simulink model "trim_cessna_t37"  (Simulink 9.0)
settings: Solver=ode45  StartTime=0.0  StopTime=10.0  RelTol=1e-3  EnableMultiTasking=on
values from neighbouring files (symbols this model uses):
  Aero_RP = Aero_RP*[-1 0 0;0 1 0;0 0 -1]    [t37_data.m]
  aileron_limits = [-0.35 0.35]*pi/180    [t37_data.m]
  CD_alpha = 0.3840    (= 0.384)    [t37_data.m]
  CD_beta = [-1.5700	1.2300 ... (first row only)    [t37_data.m]
  CD_de = 0.0750    (= 0.075)    [t37_data.m]
  CD_flap = 0.0750    (= 0.075)    [t37_data.m]
  CD_ground_effect = [0.0000	0.8100 ... (first row only)    [t37_data.m]
  CD_zero = [  -1.5700	1.5000 ... (first row only)    [t37_data.m]
  Cl_ail = [0.0000	0.1810 ... (first row only)    [t37_data.m]
  CL_alpha = [-0.2000	-0.6400 ... (first row only)    [t37_data.m]
  CL_alpha_dot = 2.0    (= 2)    [t37_data.m]
  Cl_beta = -0.0944    [t37_data.m]
  CL_elev = 0.5    [t37_data.m]
  CL_flap = 0.3500    (= 0.35)    [t37_data.m]
  CL_ground_effect = [0.0000	1.0610 ... (first row only)    [t37_data.m]
  Cl_p = -0.4420    (= -0.442)    [t37_data.m]
  CL_q = 4.1    [t37_data.m]
  Cl_r = 0.0926    [t37_data.m]
  Cl_rudder = 0.0150    (= 0.015)    [t37_data.m]
  Cm_alpha = -0.7000    (= -0.7)    [t37_data.m]
  Cm_alpha_dot = -6.9500    (= -6.95)    [t37_data.m]
  Cm_elev = [0.0000	-1.1200 ... (first row only)    [t37_data.m]
  Cm_q = -50.0000    (= -50)    [t37_data.m]
  Cm_zero = 0.0250    (= 0.025)    [t37_data.m]
  Cn_beta = 0.1106    [t37_data.m]
  Cn_p = -0.0243    [t37_data.m]
  Cn_r = -0.1390    (= -0.139)    [t37_data.m]
  Cn_rudder = -0.0365    [t37_data.m]
  Cnda = -0.0254    [t37_data.m]
  CY_beta = -0.3460    (= -0.346)    [t37_data.m]
  CY_p = -0.0827    [t37_data.m]
  CY_r = 0.3000    (= 0.3)    [t37_data.m]
  CY_rudder = 0.200    (= 0.2)    [t37_data.m]
  elevator_limits = [-0.35 0.3]*pi/180    [t37_data.m]
  isTrimming = 0    [mytrim.m]    (also in t37_data.m)
  Jxx = 7985*1.3558179    (= 10826.2059315)    [t37_data.m]
  Jxz = 0    [t37_data.m]
  Jyy = 6000*1.3558179    (= 8134.9074)    [t37_data.m]
  Jzz = 11183*1.3558179    (= 15162.1115757)    [t37_data.m]
  M = 4056*0.45359237    (= 1839.77065272)    [t37_data.m]
  Rcg = Rcg*[-1 0 0;0 1 0;0 0 -1]    [t37_data.m]
  Rengine1 = Rengine1*[-1 0 0;0 1 0;0 0 -1]    [t37_data.m]
  Rengine2 = Rengine2*[-1 0 0;0 1 0;0 0 -1]    [t37_data.m]
  rudder_limits = [-0.35 0.35]*pi/180    [t37_data.m]
  Sw = 182*0.09290304    (= 16.90835328)    [t37_data.m]
  thrust_limits = [0 1]    [t37_data.m]
  Tmax = M*10    (= 18397.7065272)    [t37_data.m]
undefined symbols (not defined in the file or in its folder): CD_mach, DCnpDf
undefined symbols (not defined in the file): Bw, Cw
libraries: sharedutil x1
(part 1 of 2)
settings Model: Creator=torres  LastModifiedBy=Pc melhor q do euler  ExtModeAutoUpdateStatusClock=off
settings DataIOCC: LimitDataPoints=on  SignalLoggingSaveFormat=ModelDataLogs  SignalLoggingName=sigsOut
settings DebuggingCC: SaveWithParameterizedLinksMsg=none  SignalResolutionControl=TryResolveAllWithWarning  MultiTaskDSMMsg=warning  MultiTaskCondExecSysMsg=none  FcnCallInpInsideContextMsg=warning  StrictBusMsg=None
settings HardwareCC: TargetHWDeviceType=32-bit Generic  TargetUnknown=on  ProdEqTarget=off
settings GRTTargetCC: TargetFcnLib=ansi_tfl_tmw.mat  CombineOutputUpdateFcns=off  GRTInterface=on

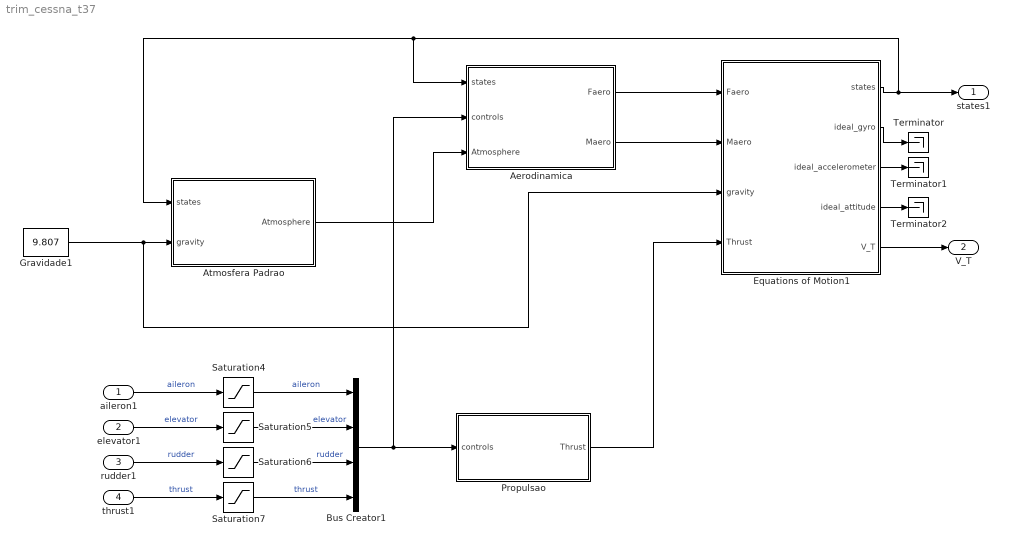
== system trim_cessna_t37 ==
  aileron1 : Inport
  elevator1 : Inport  Port=2
  rudder1 : Inport  Port=3
  thrust1 : Inport  Port=4
  Aerodinamica : Subsystem  mask{flap=0, bw=Bw, cw=Cw, Sw=Sw}
      mask prompts: flap "Comando Flap (0, 1, 2 ou 3)"; bw "Comprimento da asa  - wingspan (m)"; cw "Corda media da asa (m)"; Sw "Area da asa (m2)"
  Atmosfera Padrao : Subsystem
  Bus Creator1 : BusCreator  Inputs=4
  Equations of Motion1 : Subsystem  mask{R_engine=Rengine1, Rcg=Rcg, Aero_RP=Aero_RP, m=M, Jxz=Jxz, Jxx=Jxx, Jyy=Jyy, Jzz=Jzz, d=[0; 0; 0]}
      mask prompts: R_engine "Engine position (row vector in meters)"; Rcg "C.G. position (m)"; Aero_RP "Nominal C.G. (m) = Aerodynamic Reference Point"; m "Aircraft mass (Kg)"; Jxz "Inertia product (Jxz)"; Jxx "Inertia (Jxx)"; Jyy "Inertia (Jyy)"; Jzz "Inertia (Jzz)"; d "Accelerometers displacement from CG (vector in the ABC frame, in (m))"
  Gravidade1 : Constant  Value=9.807
  Propulsao : Subsystem  mask{Tmax=Tmax}
      mask prompts: Tmax "Tracao Maxima (N)"
  Saturation4 : Saturate  UpperLimit=aileron_limits(2)  LowerLimit=aileron_limits(1)
  Saturation5 : Saturate  UpperLimit=elevator_limits(2)  LowerLimit=elevator_limits(1)
  Saturation6 : Saturate  UpperLimit=rudder_limits(2)  LowerLimit=rudder_limits(1)
  Saturation7 : Saturate  UpperLimit=thrust_limits(2)  LowerLimit=thrust_limits(1)
  Terminator : Terminator
  Terminator1 : Terminator
  Terminator2 : Terminator
  states1 : Outport
  V_T : Outport  Port=2
  wires:
  Atmosfera Padrao/1(Atmosphere) -> Aerodinamica/3(Atmosphere)
  Equations of Motion1/1(states) -> Atmosfera Padrao/1(states), Aerodinamica/1(states), states1/1
  aileron1/1 -> Saturation4/1  "aileron"
  elevator1/1 -> Saturation5/1  "elevator"
  rudder1/1 -> Saturation6/1  "rudder"
  Gravidade1/1 -> Atmosfera Padrao/2(gravity), Equations of Motion1/3(gravity)
  thrust1/1 -> Saturation7/1  "thrust"
  Bus Creator1/1 -> Propulsao/1(controls), Aerodinamica/2(controls)
  Aerodinamica/1(Faero) -> Equations of Motion1/1(Faero)
  Aerodinamica/2(Maero) -> Equations of Motion1/2(Maero)
  Propulsao/1(Thrust) -> Equations of Motion1/4(Thrust)
  Saturation4/1 -> Bus Creator1/1  "aileron"
  Saturation5/1 -> Bus Creator1/2  "elevator"
  Saturation6/1 -> Bus Creator1/3  "rudder"
  Saturation7/1 -> Bus Creator1/4  "thrust"
  Equations of Motion1/2(ideal_gyro) -> Terminator/1
  Equations of Motion1/3(ideal_accelerometer) -> Terminator1/1
  Equations of Motion1/4(ideal_attitude) -> Terminator2/1
  Equations of Motion1/5(V_T) -> V_T/1

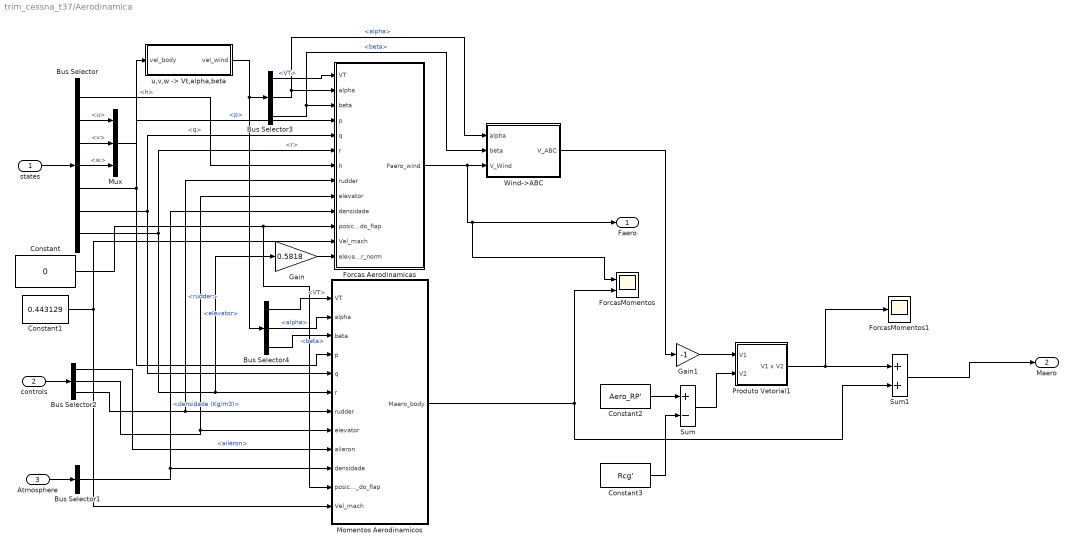
== system trim_cessna_t37/Aerodinamica ==
  states : Inport
  controls : Inport  Port=2
  Atmosphere : Inport  Port=3
  Bus Selector : BusSelector  OutputSignals=h,u,v,w,p,q,r
  Bus Selector1 : BusSelector  OutputSignals=densidade (Kg/m3)
  Bus Selector2 : BusSelector  OutputSignals=aileron,elevator,rudder
  Bus Selector3 : BusSelector  OutputSignals=VT,alpha,beta
  Bus Selector4 : BusSelector  OutputSignals=VT,alpha,beta
  Constant : Constant  Value=0
  Constant1 : Constant  Value=0.443129
  Constant2 : Constant  Value=Aero_RP'
  Constant3 : Constant  Value=Rcg'
  Forcas Aerodinamicas : Subsystem
  ForcasMomentos : Scope  NumInputPorts=2
  ForcasMomentos1 : Scope
  Gain : Gain  Gain=0.5818
  Gain1 : Gain  Gain=-1
  Momentos Aerodinamicos : Subsystem
  Mux : Mux  Inputs=3
  Produto Vetorial1 : Subsystem
  Sum : Sum  Inputs=+-  SaturateOnIntegerOverflow=on
  Sum1 : Sum  SaturateOnIntegerOverflow=on
  Wind->ABC : Subsystem
  "u,v,w -> Vt,alpha,beta" : Subsystem
  Faero : Outport
  Maero : Outport  Port=2
  wires:
  states/1 -> Bus Selector/1
  Atmosphere/1 -> Bus Selector1/1
  Bus Selector1/1 -> Momentos Aerodinamicos/10(densidade), Forcas Aerodinamicas/10(densidade)  "<densidade (Kg/m3)>"
  Bus Selector/1 -> Forcas Aerodinamicas/7(h)  "<h>"
  Bus Selector/5 -> Momentos Aerodinamicos/4(p), Forcas Aerodinamicas/4(p)  "<p>"
  Bus Selector/6 -> Momentos Aerodinamicos/5(q), Forcas Aerodinamicas/5(q)  "<q>"
  Bus Selector/7 -> Gain/1, Momentos Aerodinamicos/6(r), Forcas Aerodinamicas/6(r)  "<r>"
  controls/1 -> Bus Selector2/1
  Bus Selector2/1 -> Momentos Aerodinamicos/9(aileron)  "<aileron>"
  Bus Selector2/2 -> Momentos Aerodinamicos/8(elevator), Forcas Aerodinamicas/9(elevator)  "<elevator>"
  Bus Selector2/3 -> Momentos Aerodinamicos/7(rudder), Forcas Aerodinamicas/8(rudder)  "<rudder>"
  Bus Selector3/1 -> Forcas Aerodinamicas/1(VT)  "<VT>"
  Bus Selector3/2 -> Forcas Aerodinamicas/2(alpha), Wind->ABC/1(alpha)  "<alpha>"
  Bus Selector3/3 -> Forcas Aerodinamicas/3(beta), Wind->ABC/2(beta)  "<beta>"
  Bus Selector4/1 -> Momentos Aerodinamicos/1(VT)  "<VT>"
  Bus Selector4/2 -> Momentos Aerodinamicos/2(alpha)  "<alpha>"
  Bus Selector4/3 -> Momentos Aerodinamicos/3(beta)  "<beta>"
  "u,v,w -> Vt,alpha,beta"/1(vel_wind) -> Bus Selector3/1, Bus Selector4/1
  Bus Selector/2 -> Mux/1  "<u>"
  Bus Selector/3 -> Mux/2  "<v>"
  Bus Selector/4 -> Mux/3  "<w>"
  Mux/1 -> "u,v,w -> Vt,alpha,beta"/1(vel_body)
  Constant/1 -> Momentos Aerodinamicos/11(posicao_do_flap), Forcas Aerodinamicas/11("posicao_do_flap ")
  Constant1/1 -> Momentos Aerodinamicos/12(Vel_mach), Forcas Aerodinamicas/12(Vel_mach)
  Gain/1 -> Forcas Aerodinamicas/13(elevator_norm)
  Constant2/1 -> Sum/1
  Gain1/1 -> Produto Vetorial1/1(V1)
  Produto Vetorial1/1(V1 x V2) -> ForcasMomentos1/1, Sum1/1
  Sum1/1 -> Maero/1
  Constant3/1 -> Sum/2
  Momentos Aerodinamicos/1(Maero_body) -> Sum1/2, ForcasMomentos/2
  Sum/1 -> Produto Vetorial1/2(V2)
  Forcas Aerodinamicas/1(Faero_wind) -> ForcasMomentos/1, Faero/1, Wind->ABC/3(V_Wind)
  Wind->ABC/1(V_ABC) -> Gain1/1

== system trim_cessna_t37/Atmosfera Padrao ==
  states : Inport
  gravity : Inport  Port=2
  Bus Creator : BusCreator  Inputs=4
  Bus Selector : BusSelector  OutputSignals=h
  Calc. Densidade : Fcn  Expr=1.225*(u(1)/288.15)^(-u(2)/(-0.0065*287.04)-1)
  Calc. Pressao : Fcn  Expr=101325*(u(1)/288.15)^(-u(2)/(-0.0065*287.04))
  Calc. Temperatura : Fcn  Expr=288.15 -0.0065*u(1)
  Calc. Vel. Som : Fcn  Expr=sqrt(u*1.4*287.04)
  Mux : Mux  Inputs=2
  Mux1 : Mux  Inputs=2
  Atmosphere : Outport
  wires:
  states/1 -> Bus Selector/1
  Bus Selector/1 -> Mux/1  "<h>"
  gravity/1 -> Mux/2, Mux1/2
  Mux/1 -> Calc. Temperatura/1
  Mux1/1 -> Calc. Pressao/1, Calc. Densidade/1
  Calc. Temperatura/1 -> Mux1/1, Calc. Vel. Som/1, Bus Creator/3  "Temperatura (K)"
  Calc. Pressao/1 -> Bus Creator/4  "Pressao (Pa)"
  Calc. Densidade/1 -> Bus Creator/1  "densidade (Kg/m3)"
  Calc. Vel. Som/1 -> Bus Creator/2  "Vel_som (m/s)"
  Bus Creator/1 -> Atmosphere/1

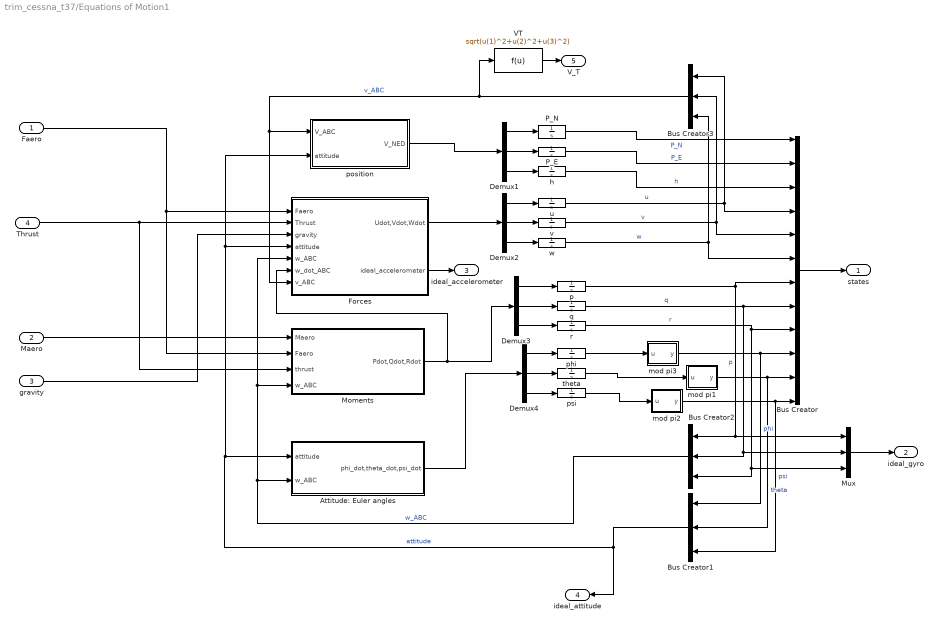
== system trim_cessna_t37/Equations of Motion1 ==
  Faero : Inport
  Maero : Inport  Port=2
  gravity : Inport  Port=3
  Thrust : Inport  Port=4
  Attitude: Euler angles : Subsystem
  Bus Creator : BusCreator  Inputs=12
  Bus Creator1 : BusCreator  Inputs=3
  Bus Creator2 : BusCreator  Inputs=3
  Bus Creator3 : BusCreator  Inputs=3
  Demux{1..4} (4 alike) : Demux  Outputs=3
  Forces : Subsystem
  Moments : Subsystem
  Mux : Mux  Inputs=3
  P_E : Integrator
  "P_N " : Integrator
  VT : Fcn  Expr=sqrt(u(1)^2+u(2)^2+u(3)^2)
  "h " : Integrator
  mod pi1 : Subsystem
  mod pi2 : Subsystem
  mod pi3 : Subsystem
  p : Integrator
  phi : Integrator
  position : Subsystem
  psi : Integrator
  q : Integrator
  r : Integrator
  theta : Integrator
  u : Integrator
  v : Integrator
  w : Integrator
  states : Outport
  ideal_gyro : Outport  Port=2
  ideal_accelerometer : Outport  Port=3
  ideal_attitude : Outport  Port=4
  V_T : Outport  Port=5
  wires:
  "h "/1 -> Bus Creator/3  "h"
  u/1 -> Bus Creator/4, Bus Creator3/1  "u"
  v/1 -> Bus Creator/5, Bus Creator3/2  "v"
  w/1 -> Bus Creator/6, Bus Creator3/3  "w"
  p/1 -> Bus Creator/7, Bus Creator2/1, Mux/1  "p"
  q/1 -> Bus Creator/8, Bus Creator2/2, Mux/2  "q"
  r/1 -> Bus Creator/9, Bus Creator2/3, Mux/3  "r"
  phi/1 -> mod pi3/1(u)
  theta/1 -> mod pi1/1(u)
  psi/1 -> mod pi2/1(u)
  Bus Creator/1 -> states/1
  Thrust/1 -> Moments/3(thrust), Forces/2(Thrust)
  Bus Creator1/1 -> Attitude: Euler angles/1(attitude), Forces/4(attitude), position/2(attitude), ideal_attitude/1  "attitude"
  Forces/1(Udot,Vdot,Wdot) -> Demux2/1
  gravity/1 -> Forces/3(gravity)
  Attitude: Euler angles/1(phi_dot,theta_dot,psi_dot) -> Demux4/1
  Maero/1 -> Moments/1(Maero)
  Bus Creator3/1 -> VT/1, Forces/7(v_ABC), position/1(V_ABC)  "v_ABC"
  Faero/1 -> Moments/2(Faero), Forces/1(Faero)
  Bus Creator2/1 -> Attitude: Euler angles/2(w_ABC), Moments/4(w_ABC), Forces/5(w_ABC)  "w_ABC"
  Moments/1(Pdot,Qdot,Rdot) -> Demux3/1, Forces/6(w_dot_ABC)
  "P_N "/1 -> Bus Creator/1  "P_N"
  P_E/1 -> Bus Creator/2  "P_E"
  position/1(V_NED) -> Demux1/1
  mod pi3/1(y) -> Bus Creator/10, Bus Creator1/1  "phi"
  mod pi1/1(y) -> Bus Creator/11, Bus Creator1/2  "theta"
  mod pi2/1(y) -> Bus Creator/12, Bus Creator1/3  "psi"
  Mux/1 -> ideal_gyro/1
  Forces/2(ideal_accelerometer) -> ideal_accelerometer/1
  VT/1 -> V_T/1
  Demux1/2 -> P_E/1
  Demux1/1 -> "P_N "/1
  Demux1/3 -> "h "/1
  Demux2/1 -> u/1
  Demux2/2 -> v/1
  Demux2/3 -> w/1
  Demux3/1 -> p/1
  Demux3/2 -> q/1
  Demux3/3 -> r/1
  Demux4/1 -> phi/1
  Demux4/2 -> theta/1
  Demux4/3 -> psi/1

== system trim_cessna_t37/Propulsao ==
  controls : Inport
  Bus Selector : BusSelector  OutputSignals=thrust
  Constant : Constant  Value=0
  Gain : Gain  Gain=Tmax  SaturateOnIntegerOverflow=on  OutDataTypeStr=Inherit: Same as input  ParamDataTypeStr=Inherit: Same as input
  Mux : Mux  Inputs=3
  Saturation : Saturate  UpperLimit=1  LowerLimit=0.0
  Thrust : Outport
  wires:
  Saturation/1 -> Gain/1
  controls/1 -> Bus Selector/1
  Bus Selector/1 -> Saturation/1  "<thrust>"
  Gain/1 -> Mux/1
  Mux/1 -> Thrust/1
  Constant/1 -> Mux/3, Mux/2

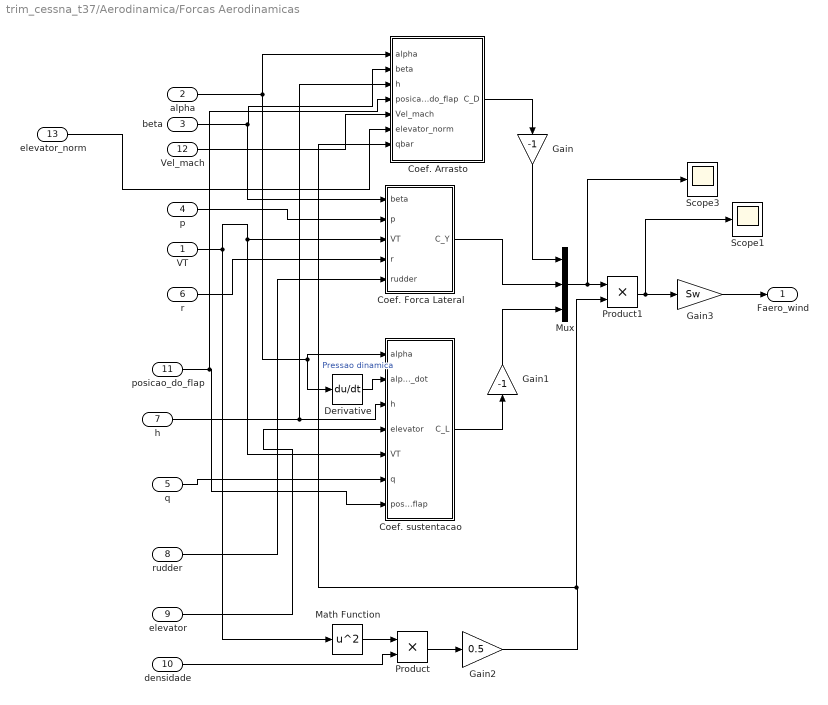
== system trim_cessna_t37/Aerodinamica/Forcas Aerodinamicas ==
  VT : Inport
  alpha : Inport  Port=2
  beta : Inport  Port=3
  p : Inport  Port=4
  q : Inport  Port=5
  r : Inport  Port=6
  h : Inport  Port=7
  rudder : Inport  Port=8
  elevator : Inport  Port=9
  densidade : Inport  Port=10
  "posicao_do_flap " : Inport  Port=11
  Vel_mach : Inport  Port=12
  elevator_norm : Inport  Port=13
  Coef. Arrasto : Subsystem
  Coef. Forca Lateral : Subsystem
  Coef. sustentacao : Subsystem
  Derivative : Derivative
  Gain : Gain  Gain=-1  SaturateOnIntegerOverflow=on  OutDataTypeStr=Inherit: Same as input  ParamDataTypeStr=Inherit: Same as input
  Gain1 : Gain  Gain=-1  SaturateOnIntegerOverflow=on  OutDataTypeStr=Inherit: Same as input  ParamDataTypeStr=Inherit: Same as input
  Gain2 : Gain  Gain=0.5  SaturateOnIntegerOverflow=on  OutDataTypeStr=Inherit: Same as input  ParamDataTypeStr=Inherit: Same as input
  Gain3 : Gain  Gain=Sw  SaturateOnIntegerOverflow=on  OutDataTypeStr=Inherit: Same as input  ParamDataTypeStr=Inherit: Same as input
  Math Function : Math  Operator=square  SaturateOnIntegerOverflow=on
  Mux : Mux  Inputs=3
  Product : Product  SaturateOnIntegerOverflow=on  OutDataTypeStr=Inherit: Same as first input
  Product1 : Product  SaturateOnIntegerOverflow=on  OutDataTypeStr=Inherit: Same as first input
  Scope1 : Scope
  Scope3 : Scope
  Faero_wind : Outport
  wires:
  Coef. Arrasto/1(C_D) -> Gain/1
  Coef. Forca Lateral/1(C_Y) -> Mux/2
  alpha/1 -> Coef. Arrasto/1(alpha), Coef. sustentacao/1(alpha), Derivative/1
  beta/1 -> Coef. Arrasto/2(beta), Coef. Forca Lateral/1(beta)
  VT/1 -> Coef. Forca Lateral/3(VT), Coef. sustentacao/5(VT), Math Function/1
  p/1 -> Coef. Forca Lateral/2(p)
  q/1 -> Coef. sustentacao/6(q)
  r/1 -> Coef. Forca Lateral/4(r)
  h/1 -> Coef. Arrasto/3(h), Coef. sustentacao/3(h)
  rudder/1 -> Coef. Forca Lateral/5(rudder)
  elevator/1 -> Coef. sustentacao/4(elevator)
  Derivative/1 -> Coef. sustentacao/2(alpha_dot)
  Coef. sustentacao/1(C_L) -> Gain1/1
  Gain/1 -> Mux/1
  Gain1/1 -> Mux/3
  densidade/1 -> Product/2
  Math Function/1 -> Product/1
  Product/1 -> Gain2/1
  Mux/1 -> Scope3/1, Product1/1
  Product1/1 -> Scope1/1, Gain3/1
  Gain2/1 -> Product1/2, Coef. Arrasto/7(qbar)  "Pressao dinamica"
  Gain3/1 -> Faero_wind/1
  "posicao_do_flap "/1 -> Coef. Arrasto/4(posicao_do_flap), Coef. sustentacao/7("posicao_do_flap ")
  Vel_mach/1 -> Coef. Arrasto/5(Vel_mach)
  elevator_norm/1 -> Coef. Arrasto/6(elevator_norm)

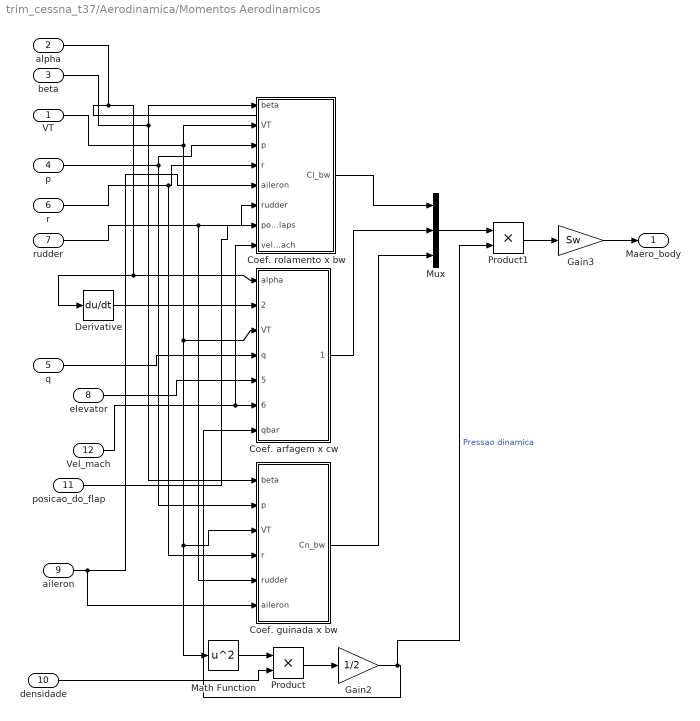
== system trim_cessna_t37/Aerodinamica/Momentos Aerodinamicos ==
  VT : Inport
  alpha : Inport  Port=2
  beta : Inport  Port=3
  p : Inport  Port=4
  q : Inport  Port=5
  r : Inport  Port=6
  rudder : Inport  Port=7
  elevator : Inport  Port=8
  aileron : Inport  Port=9
  densidade : Inport  Port=10
  posicao_do_flap : Inport  Port=11
  Vel_mach : Inport  Port=12
  Coef. arfagem x cw : Subsystem
  Coef. guinada x bw : Subsystem
  Coef. rolamento x bw : Subsystem
  Derivative : Derivative
  Gain2 : Gain  Gain=1/2  SaturateOnIntegerOverflow=on  OutDataTypeStr=Inherit: Same as input  ParamDataTypeStr=Inherit: Same as input
  Gain3 : Gain  Gain=Sw  SaturateOnIntegerOverflow=on  OutDataTypeStr=Inherit: Same as input  ParamDataTypeStr=Inherit: Same as input
  Math Function : Math  Operator=square  SaturateOnIntegerOverflow=on
  Mux : Mux  Inputs=3
  Product : Product  SaturateOnIntegerOverflow=on  OutDataTypeStr=Inherit: Same as first input
  Product1 : Product  SaturateOnIntegerOverflow=on  OutDataTypeStr=Inherit: Same as first input
  Maero_body : Outport
  wires:
  alpha/1 -> Coef. arfagem x cw/1(alpha), Derivative/1
  beta/1 -> Coef. guinada x bw/1(beta), Coef. rolamento x bw/1(beta)
  VT/1 -> Coef. arfagem x cw/3(VT), Coef. guinada x bw/3(VT), Math Function/1, Coef. rolamento x bw/2(VT)
  p/1 -> Coef. rolamento x bw/3(p), Coef. guinada x bw/2(p)
  r/1 -> Coef. rolamento x bw/4(r), Coef. guinada x bw/4(r)
  Derivative/1 -> Coef. arfagem x cw/2(alpha_dot)
  q/1 -> Coef. arfagem x cw/4(q)
  rudder/1 -> Coef. rolamento x bw/6(rudder), Coef. guinada x bw/5(rudder)
  elevator/1 -> Coef. arfagem x cw/5(elevator)
  aileron/1 -> Coef. guinada x bw/6("aileron "), Coef. rolamento x bw/5(aileron)
  Mux/1 -> Product1/1
  Product1/1 -> Gain3/1
  Coef. rolamento x bw/1(Cl_bw) -> Mux/1
  Coef. arfagem x cw/1(Cm_cw) -> Mux/2
  Coef. guinada x bw/1(Cn_bw) -> Mux/3
  densidade/1 -> Product/2
  Math Function/1 -> Product/1
  Product/1 -> Gain2/1
  Gain2/1 -> Product1/2, Coef. arfagem x cw/7(qbar)  "Pressao dinamica"
  Gain3/1 -> Maero_body/1
  posicao_do_flap/1 -> Coef. rolamento x bw/7(posicao_dos_flaps)
  Vel_mach/1 -> Coef. rolamento x bw/8(vel_mach), Coef. arfagem x cw/6(Vel_mach)

== system trim_cessna_t37/Aerodinamica/Produto Vetorial1 ==
  V1 : Inport
  V2 : Inport  Port=2
  3x3 Cross Product : sharedutil/3x3 Cross Product
      settings: SourceProductBaseCode=AE
  V1 x V2 : Outport
  wires:
  V1/1 -> 3x3 Cross Product/1
  V2/1 -> 3x3 Cross Product/2
  3x3 Cross Product/1 -> V1 x V2/1

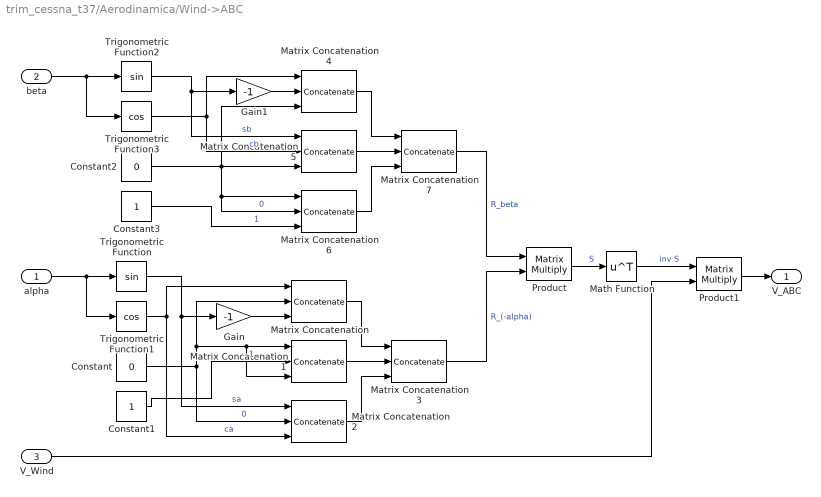
== system trim_cessna_t37/Aerodinamica/Wind->ABC ==
  alpha : Inport
  beta : Inport  Port=2
  V_Wind : Inport  Port=3
  Constant : Constant  Value=0
  Constant1 : Constant
  Constant2 : Constant  Value=0
  Constant3 : Constant
  Gain : Gain  Gain=-1  SaturateOnIntegerOverflow=on  OutDataTypeStr=Inherit: Same as input  ParamDataTypeStr=Inherit: Same as input
  Gain1 : Gain  Gain=-1  SaturateOnIntegerOverflow=on  OutDataTypeStr=Inherit: Same as input  ParamDataTypeStr=Inherit: Same as input
  Math Function : Math  Operator=transpose  SaturateOnIntegerOverflow=on
  Matrix Concatenation{,1..2,4..6} (6 alike) : Concatenate  NumInputs=3  Mode=Multidimensional array
  Matrix Concatenation3 : Concatenate  NumInputs=3  Mode=Multidimensional array  ConcatenateDimension=2
  Matrix Concatenation7 : Concatenate  NumInputs=3  Mode=Multidimensional array  ConcatenateDimension=2
  Product : Product  Multiplication=Matrix(*)  SaturateOnIntegerOverflow=on  OutDataTypeStr=Inherit: Same as first input
  Product1 : Product  Multiplication=Matrix(*)  SaturateOnIntegerOverflow=on  OutDataTypeStr=Inherit: Same as first input
  Trigonometric Function : Trigonometry
  Trigonometric Function1 : Trigonometry  Operator=cos
  Trigonometric Function2 : Trigonometry
  Trigonometric Function3 : Trigonometry  Operator=cos
  V_ABC : Outport
  wires:
  alpha/1 -> Trigonometric Function/1, Trigonometric Function1/1
  Trigonometric Function1/1 -> Matrix Concatenation/1, Matrix Concatenation2/3  "ca"
  Trigonometric Function/1 -> Matrix Concatenation2/1, Gain/1  "sa"
  Constant/1 -> Matrix Concatenation/2, Matrix Concatenation1/1, Matrix Concatenation1/3, Matrix Concatenation2/2  "0"
  Constant1/1 -> Matrix Concatenation1/2  "1"
  Matrix Concatenation/1 -> Matrix Concatenation3/1
  Matrix Concatenation1/1 -> Matrix Concatenation3/2
  Matrix Concatenation2/1 -> Matrix Concatenation3/3
  Product/1 -> Math Function/1  "S"
  Math Function/1 -> Product1/1  "inv S"
  Product1/1 -> V_ABC/1
  beta/1 -> Trigonometric Function2/1, Trigonometric Function3/1
  Matrix Concatenation4/1 -> Matrix Concatenation7/1
  Matrix Concatenation5/1 -> Matrix Concatenation7/2
  Matrix Concatenation6/1 -> Matrix Concatenation7/3
  Trigonometric Function3/1 -> Matrix Concatenation4/1, Matrix Concatenation5/2  "cb"
  Trigonometric Function2/1 -> Gain1/1, Matrix Concatenation5/1  "sb"
  Constant2/1 -> Matrix Concatenation4/3, Matrix Concatenation5/3, Matrix Concatenation6/1, Matrix Concatenation6/2  "0"
  Constant3/1 -> Matrix Concatenation6/3  "1"
  Matrix Concatenation7/1 -> Product/1  "R_beta"
  Matrix Concatenation3/1 -> Product/2  "R_(-alpha)"
  Gain1/1 -> Matrix Concatenation4/2
  V_Wind/1 -> Product1/2
  Gain/1 -> Matrix Concatenation/3

== system trim_cessna_t37/Aerodinamica/u,v,w -> Vt,alpha,beta ==
  vel_body : Inport
  Bus Creator : BusCreator  Inputs=3
  VT : Fcn  Expr=sqrt(u(1)^2+u(2)^2+u(3)^2)
  alpha : Fcn  Expr=atan2(u(3),u(1))
  beta : Fcn  Expr=atan2(u(2),sqrt(u(1)^2+u(3)^2))
  vel_wind : Outport
  wires:
  Bus Creator/1 -> vel_wind/1
  VT/1 -> Bus Creator/1  "VT"
  alpha/1 -> Bus Creator/2  "alpha"
  vel_body/1 -> alpha/1, VT/1, beta/1
  beta/1 -> Bus Creator/3  "beta"

== system trim_cessna_t37/Equations of Motion1/Attitude: Euler angles ==
  attitude : Inport
  w_ABC : Inport  Port=2
  Bus Selector : BusSelector  OutputSignals=phi,theta,psi
  Bus Selector1 : BusSelector  OutputSignals=p,q,r
  Mux : Mux  Inputs=3
  Product{,1..4,6..7} (7 alike) : Product  SaturateOnIntegerOverflow=on  OutDataTypeStr=Inherit: Same as first input
  Product5 : Product  Inputs=/*  SaturateOnIntegerOverflow=on  OutDataTypeStr=Inherit: Same as first input
  Sum1 : Sum  SaturateOnIntegerOverflow=on
  Sum2 : Sum  SaturateOnIntegerOverflow=on
  Sum3 : Sum  Inputs=+-  SaturateOnIntegerOverflow=on
  Sum4 : Sum  SaturateOnIntegerOverflow=on
  Terminator : Terminator
  Trigonometric Function : Trigonometry  Operator=tan
  Trigonometric Function1 : Trigonometry
  Trigonometric Function2 : Trigonometry  Operator=cos
  Trigonometric Function3 : Trigonometry  Operator=cos
  phi_dot,theta_dot,psi_dot : Outport
  wires:
  Bus Selector/2 -> Trigonometric Function3/1, Trigonometric Function/1  "<theta>"
  Bus Selector/1 -> Trigonometric Function1/1, Trigonometric Function2/1  "<phi>"
  Trigonometric Function1/1 -> Product/1, Product4/1, Product6/1
  Trigonometric Function2/1 -> Product1/1, Product3/1, Product7/1
  Product1/1 -> Sum1/1
  Product/1 -> Sum1/2
  Sum1/1 -> Product2/1
  Product2/1 -> Sum2/1
  Sum2/1 -> Mux/1
  attitude/1 -> Bus Selector/1
  Bus Selector/3 -> Terminator/1  "<psi>"
  Product3/1 -> Sum3/1
  w_ABC/1 -> Bus Selector1/1
  Product4/1 -> Sum3/2
  Trigonometric Function3/1 -> Product5/1
  Product6/1 -> Sum4/1
  Product7/1 -> Sum4/2
  Sum4/1 -> Product5/2
  Sum3/1 -> Mux/2
  Product5/1 -> Mux/3
  Bus Selector1/1 -> Sum2/2  "<p>"
  Mux/1 -> phi_dot,theta_dot,psi_dot/1
  Bus Selector1/2 -> Product/2, Product3/2, Product6/2  "<q>"
  Bus Selector1/3 -> Product1/2, Product4/2, Product7/2  "<r>"
  Trigonometric Function/1 -> Product2/2

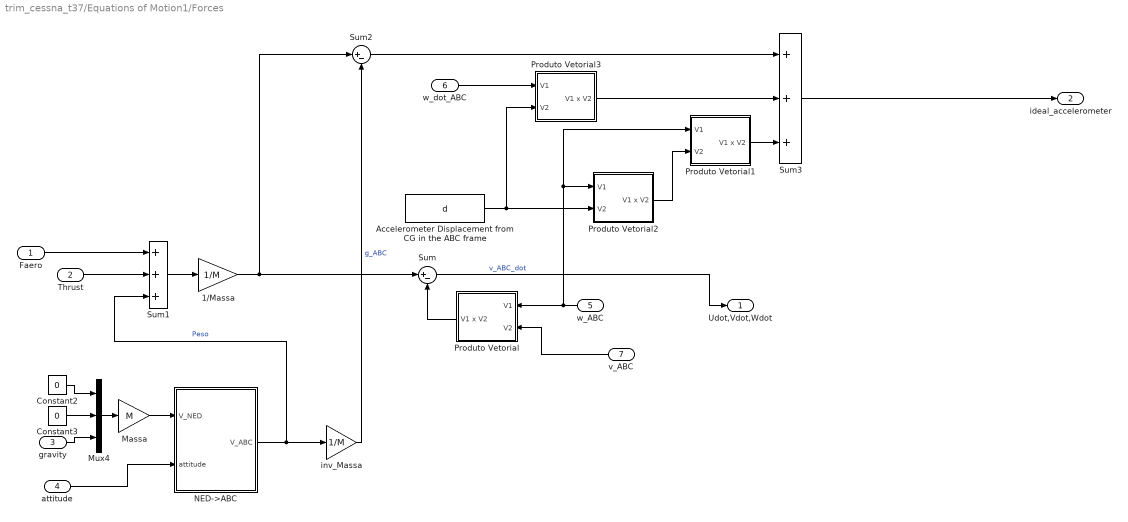
== system trim_cessna_t37/Equations of Motion1/Forces ==
  Faero : Inport
  Thrust : Inport  Port=2
  gravity : Inport  Port=3
  attitude : Inport  Port=4
  w_ABC : Inport  Port=5
  w_dot_ABC : Inport  Port=6
  v_ABC : Inport  Port=7
  1/Massa : Gain  Gain=1/M  SaturateOnIntegerOverflow=on  OutDataTypeStr=Inherit: Same as input  ParamDataTypeStr=Inherit: Same as input
  Accelerometer Displacement from CG in the ABC frame : Constant  Value=d
  Constant2 : Constant  Value=0
  Constant3 : Constant  Value=0
  Massa : Gain  Gain=M  SaturateOnIntegerOverflow=on  OutDataTypeStr=Inherit: Same as input  ParamDataTypeStr=Inherit: Same as input
  Mux4 : Mux  Inputs=3
  NED->ABC : Subsystem
  Produto Vetorial : Subsystem
  Produto Vetorial1 : Subsystem
  Produto Vetorial2 : Subsystem
  Produto Vetorial3 : Subsystem
  Sum : Sum  Inputs=|+-  SaturateOnIntegerOverflow=on
  Sum1 : Sum  Inputs=+++  SaturateOnIntegerOverflow=on
  Sum2 : Sum  Inputs=|+-  SaturateOnIntegerOverflow=on
  Sum3 : Sum  Inputs=+++  SaturateOnIntegerOverflow=on
  inv_Massa : Gain  Gain=1/M  SaturateOnIntegerOverflow=on  OutDataTypeStr=Inherit: Same as input  ParamDataTypeStr=Inherit: Same as input
  Udot,Vdot,Wdot : Outport
  ideal_accelerometer : Outport  Port=2
  wires:
  1/Massa/1 -> Sum/1, Sum2/1
  Produto Vetorial/1(V1 x V2) -> Sum/2
  w_ABC/1 -> Produto Vetorial/1(V1), Produto Vetorial2/1(V1), Produto Vetorial1/1(V1)
  v_ABC/1 -> Produto Vetorial/2(V2)
  Sum1/1 -> 1/Massa/1
  Constant2/1 -> Mux4/1
  Constant3/1 -> Mux4/2
  gravity/1 -> Mux4/3
  Mux4/1 -> Massa/1
  Massa/1 -> NED->ABC/1(V_NED)
  attitude/1 -> NED->ABC/2(attitude)
  Faero/1 -> Sum1/1
  Thrust/1 -> Sum1/2
  Sum/1 -> Udot,Vdot,Wdot/1  "v_ABC_dot"
  NED->ABC/1(V_ABC) -> Sum1/3, inv_Massa/1  "Peso"
  inv_Massa/1 -> Sum2/2  "g_ABC"
  Sum2/1 -> Sum3/1
  Sum3/1 -> ideal_accelerometer/1
  Produto Vetorial2/1(V1 x V2) -> Produto Vetorial1/2(V2)
  Accelerometer Displacement from CG in the ABC frame/1 -> Produto Vetorial2/2(V2), Produto Vetorial3/2(V2)
  Produto Vetorial1/1(V1 x V2) -> Sum3/3
  Produto Vetorial3/1(V1 x V2) -> Sum3/2
  w_dot_ABC/1 -> Produto Vetorial3/1(V1)

== system trim_cessna_t37/Equations of Motion1/Moments ==
  Maero : Inport
  Faero : Inport  Port=2
  thrust : Inport  Port=3
  w_ABC : Inport  Port=4
  Aerodynamic Forces  point of application : Constant  Value=Aero_RP
  C.G. position : Constant  Value=Rcg
  Engine position : Constant  Value=Rengine1
  Engine position 2 : Constant  Value=Rengine2
  Inertia : Subsystem
  Inverse Inertia Matrix : Subsystem
  Product : Product  Multiplication=Matrix(*)  SaturateOnIntegerOverflow=on  OutDataTypeStr=Inherit: Same as first input
  Product1 : Product  Multiplication=Matrix(*)  SaturateOnIntegerOverflow=on  OutDataTypeStr=Inherit: Same as first input
  Product2 : Product  Multiplication=Matrix(*)  SaturateOnIntegerOverflow=on  OutDataTypeStr=Inherit: Same as first input
  Produto Vetorial1 : Subsystem
  Produto Vetorial2 : Subsystem
  Produto Vetorial3 : Subsystem
  Produto Vetorial4 : Subsystem
  Sum1 : Sum  Inputs=|+-  SaturateOnIntegerOverflow=on
  Sum2 : Sum  Inputs=++++  SaturateOnIntegerOverflow=on
  Sum3 : Sum  Inputs=|+-  SaturateOnIntegerOverflow=on
  Sum4 : Sum  Inputs=|-+  SaturateOnIntegerOverflow=on
  Sum5 : Sum  Inputs=|+-  SaturateOnIntegerOverflow=on
  Pdot,Qdot,Rdot : Outport
  wires:
  Sum2/1 -> Product/2
  Aerodynamic Forces  point of application/1 -> Sum4/2
  Product/1 -> Sum3/1
  Faero/1 -> Produto Vetorial3/2(V2)
  Inertia/1(J) -> Product1/1
  Inverse Inertia Matrix/1(inv J) -> Product/1, Product2/1
  Product2/1 -> Sum3/2
  Sum4/1 -> Produto Vetorial3/1(V1)
  Produto Vetorial1/1(V1 x V2) -> Product2/2
  C.G. position/1 -> Sum5/2, Sum1/2, Sum4/1
  Product1/1 -> Produto Vetorial1/2(V2)
  w_ABC/1 -> Product1/2, Produto Vetorial1/1(V1)
  Produto Vetorial4/1(V1 x V2) -> Sum2/4
  Produto Vetorial2/1(V1 x V2) -> Sum2/2
  Produto Vetorial3/1(V1 x V2) -> Sum2/3
  Engine position 2/1 -> Sum1/1
  Maero/1 -> Sum2/1
  Sum5/1 -> Produto Vetorial2/1(V1)
  Sum3/1 -> Pdot,Qdot,Rdot/1
  Engine position/1 -> Sum5/1
  thrust/1 -> Produto Vetorial4/2(V2), Produto Vetorial2/2(V2)
  Sum1/1 -> Produto Vetorial4/1(V1)

== system trim_cessna_t37/Equations of Motion1/mod pi1 ==
  u : Inport
  Abs : Abs  SaturateOnIntegerOverflow=on
  Constant : Constant  Value=pi
  Fcn : Fcn  Expr=u/pi
  Fcn1 : Fcn  Expr=u*pi
  Gain : Gain  Gain=1/2  SaturateOnIntegerOverflow=on  OutDataTypeStr=Inherit: Same as input  ParamDataTypeStr=Inherit: Same as input
  Gain1 : Gain  Gain=2  SaturateOnIntegerOverflow=on  OutDataTypeStr=Inherit: Same as input  ParamDataTypeStr=Inherit: Same as input
  Product : Product  SaturateOnIntegerOverflow=on  OutDataTypeStr=Inherit: Same as first input
  Rounding Function : Rounding  Operator=fix
  Rounding Function1 : Rounding  Operator=fix
  Sign : Signum
  Sum : Sum  Inputs=|-+  SaturateOnIntegerOverflow=on
  Sum1 : Sum  Inputs=-+|  SaturateOnIntegerOverflow=on
  Sum2 : Sum  Inputs=+-|  SaturateOnIntegerOverflow=on
  Switch1 : Switch  Threshold=0.5  SaturateOnIntegerOverflow=on
  y : Outport
  wires:
  u/1 -> Abs/1, Sign/1
  Fcn/1 -> Rounding Function/1
  Rounding Function/1 -> Fcn1/1, Gain/1, Sum2/1
  Fcn1/1 -> Sum/1
  Abs/1 -> Fcn/1, Sum/2
  Sign/1 -> Product/2
  Product/1 -> y/1
  Sum/1 -> Sum1/2, Switch1/3
  Constant/1 -> Sum1/1
  Sum1/1 -> Switch1/1
  Switch1/1 -> Product/1
  Gain/1 -> Rounding Function1/1
  Rounding Function1/1 -> Gain1/1
  Gain1/1 -> Sum2/2
  Sum2/1 -> Switch1/2

== system trim_cessna_t37/Equations of Motion1/mod pi2 ==
  u : Inport
  Abs : Abs  SaturateOnIntegerOverflow=on
  Constant : Constant  Value=pi
  Fcn : Fcn  Expr=u/pi
  Fcn1 : Fcn  Expr=u*pi
  Gain : Gain  Gain=1/2  SaturateOnIntegerOverflow=on  OutDataTypeStr=Inherit: Same as input  ParamDataTypeStr=Inherit: Same as input
  Gain1 : Gain  Gain=2  SaturateOnIntegerOverflow=on  OutDataTypeStr=Inherit: Same as input  ParamDataTypeStr=Inherit: Same as input
  Product : Product  SaturateOnIntegerOverflow=on  OutDataTypeStr=Inherit: Same as first input
  Rounding Function : Rounding  Operator=fix
  Rounding Function1 : Rounding  Operator=fix
  Sign : Signum
  Sum : Sum  Inputs=|-+  SaturateOnIntegerOverflow=on
  Sum1 : Sum  Inputs=-+|  SaturateOnIntegerOverflow=on
  Sum2 : Sum  Inputs=+-|  SaturateOnIntegerOverflow=on
  Switch1 : Switch  Threshold=0.5  SaturateOnIntegerOverflow=on
  y : Outport
  wires:
  u/1 -> Abs/1, Sign/1
  Fcn/1 -> Rounding Function/1
  Rounding Function/1 -> Fcn1/1, Gain/1, Sum2/1
  Fcn1/1 -> Sum/1
  Abs/1 -> Fcn/1, Sum/2
  Sign/1 -> Product/2
  Product/1 -> y/1
  Sum/1 -> Sum1/2, Switch1/3
  Constant/1 -> Sum1/1
  Sum1/1 -> Switch1/1
  Switch1/1 -> Product/1
  Gain/1 -> Rounding Function1/1
  Rounding Function1/1 -> Gain1/1
  Gain1/1 -> Sum2/2
  Sum2/1 -> Switch1/2

== system trim_cessna_t37/Equations of Motion1/mod pi3 ==
  u : Inport
  Abs : Abs  SaturateOnIntegerOverflow=on
  Constant : Constant  Value=pi
  Fcn : Fcn  Expr=u/pi
  Fcn1 : Fcn  Expr=u*pi
  Gain : Gain  Gain=1/2  SaturateOnIntegerOverflow=on  OutDataTypeStr=Inherit: Same as input  ParamDataTypeStr=Inherit: Same as input
  Gain1 : Gain  Gain=2  SaturateOnIntegerOverflow=on  OutDataTypeStr=Inherit: Same as input  ParamDataTypeStr=Inherit: Same as input
  Product : Product  SaturateOnIntegerOverflow=on  OutDataTypeStr=Inherit: Same as first input
  Rounding Function : Rounding  Operator=fix
  Rounding Function1 : Rounding  Operator=fix
  Sign : Signum
  Sum : Sum  Inputs=|-+  SaturateOnIntegerOverflow=on
  Sum1 : Sum  Inputs=-+|  SaturateOnIntegerOverflow=on
  Sum2 : Sum  Inputs=+-|  SaturateOnIntegerOverflow=on
  Switch1 : Switch  Threshold=0.5  SaturateOnIntegerOverflow=on
  y : Outport
  wires:
  u/1 -> Abs/1, Sign/1
  Fcn/1 -> Rounding Function/1
  Rounding Function/1 -> Fcn1/1, Gain/1, Sum2/1
  Fcn1/1 -> Sum/1
  Abs/1 -> Fcn/1, Sum/2
  Sign/1 -> Product/2
  Product/1 -> y/1
  Sum/1 -> Sum1/2, Switch1/3
  Constant/1 -> Sum1/1
  Sum1/1 -> Switch1/1
  Switch1/1 -> Product/1
  Gain/1 -> Rounding Function1/1
  Rounding Function1/1 -> Gain1/1
  Gain1/1 -> Sum2/2
  Sum2/1 -> Switch1/2

== system trim_cessna_t37/Equations of Motion1/position ==
  V_ABC : Inport
  attitude : Inport  Port=2
  ABC->NED : Subsystem
  Constant : Constant  Value=0  VectorParams1D=off
  Constant1 : Constant  Value=isTrimming  VectorParams1D=off
  Demux1 : Demux  Outputs=3
  Gain : Gain  Gain=-1  SaturateOnIntegerOverflow=on  OutDataTypeStr=Inherit: Same as input  ParamDataTypeStr=Inherit: Same as input
  Mux : Mux  Inputs=3
  Switch : Switch  Threshold=0.5  SaturateOnIntegerOverflow=on
  Switch1 : Switch  Threshold=0.5  SaturateOnIntegerOverflow=on
  V_NED : Outport
  wires:
  ABC->NED/1(V_NED) -> Demux1/1
  V_ABC/1 -> ABC->NED/1(V_ABC)
  attitude/1 -> ABC->NED/2(attitude)
  Demux1/3 -> Gain/1  "-h"
  Gain/1 -> Mux/3
  Mux/1 -> V_NED/1
  Switch/1 -> Mux/1
  Demux1/1 -> Switch/3  "V_N"
  Switch1/1 -> Mux/2
  Demux1/2 -> Switch1/3  "V_E"
  Constant/1 -> Switch/1, Switch1/1
  Constant1/1 -> Switch/2, Switch1/2

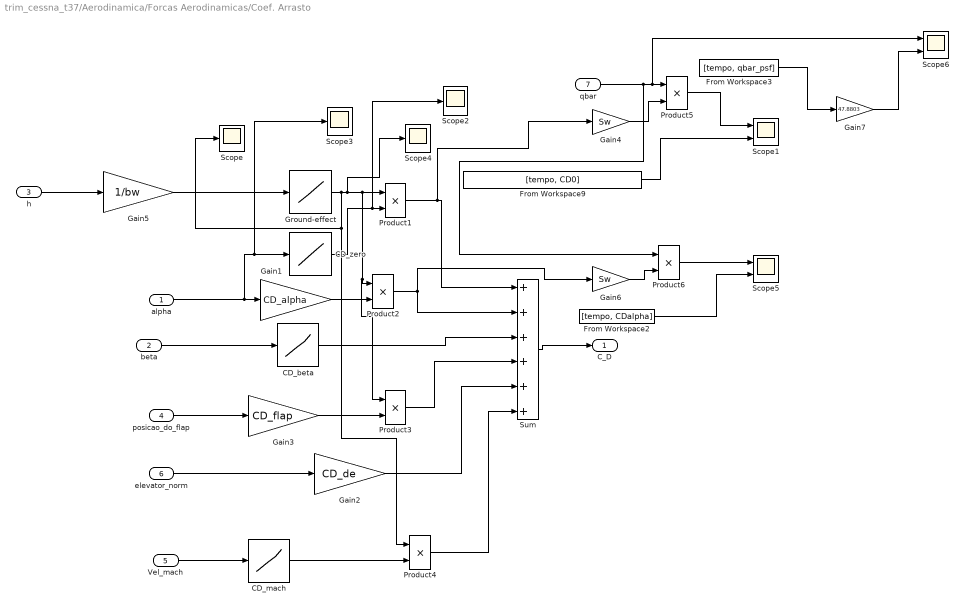
== system trim_cessna_t37/Aerodinamica/Forcas Aerodinamicas/Coef. Arrasto ==
  alpha : Inport
  beta : Inport  Port=2
  h : Inport  Port=3
  posicao_do_flap : Inport  Port=4
  Vel_mach : Inport  Port=5
  elevator_norm : Inport  Port=6
  qbar : Inport  Port=7
  CD_beta : Lookup  InputValues=CD_beta(:,1);  Table=CD_beta(:,2);  SaturateOnIntegerOverflow=on
  CD_mach : Lookup  InputValues=CD_mach(:,1);  Table=CD_mach(:,2);  SaturateOnIntegerOverflow=on
  CD_zero : Lookup  InputValues=CD_zero(:,1);  Table=CD_zero(:,2);  LookUpMeth=Interpolation-Use End Values  SaturateOnIntegerOverflow=on
  From Workspace2 : FromWorkspace  VariableName=[tempo, CDalpha]  SampleTime=0
  From Workspace3 : FromWorkspace  VariableName=[tempo, qbar_psf]  SampleTime=0
  From Workspace9 : FromWorkspace  VariableName=[tempo, CD0]  SampleTime=0
  Gain1 : Gain  Gain=CD_alpha  SaturateOnIntegerOverflow=on  OutDataTypeStr=Inherit: Same as input  ParamDataTypeStr=Inherit: Same as input
  Gain2 : Gain  Gain=CD_de  SaturateOnIntegerOverflow=on  OutDataTypeStr=Inherit: Same as input  ParamDataTypeStr=Inherit: Same as input
  Gain3 : Gain  Gain=CD_flap  SaturateOnIntegerOverflow=on  OutDataTypeStr=Inherit: Same as input  ParamDataTypeStr=Inherit: Same as input
  Gain4 : Gain  Gain=Sw  SaturateOnIntegerOverflow=on  OutDataTypeStr=Inherit: Same as input  ParamDataTypeStr=Inherit: Same as input
  Gain5 : Gain  Gain=1/bw  SaturateOnIntegerOverflow=on  OutDataTypeStr=Inherit: Same as input  ParamDataTypeStr=Inherit: Same as input
  Gain6 : Gain  Gain=Sw  SaturateOnIntegerOverflow=on  OutDataTypeStr=Inherit: Same as input  ParamDataTypeStr=Inherit: Same as input
  Gain7 : Gain  Gain=47.8803  SaturateOnIntegerOverflow=on  OutDataTypeStr=Inherit: Same as input  ParamDataTypeStr=Inherit: Same as input
  Ground-effect : Lookup  InputValues=CD_ground_effect(:,1);  Table=CD_ground_effect(:,2);  LookUpMeth=Interpolation-Use End Values  SaturateOnIntegerOverflow=on
  Product{1..6} (6 alike) : Product  SaturateOnIntegerOverflow=on  OutDataTypeStr=Inherit: Same as first input
  Scope{,2..4} (4 alike) : Scope
  Scope1 : Scope  NumInputPorts=2
  Scope5 : Scope  NumInputPorts=2
  Scope6 : Scope  NumInputPorts=2
  Sum : Sum  Inputs=++++++  SaturateOnIntegerOverflow=on
  C_D : Outport
  wires:
  alpha/1 -> Gain1/1, Scope3/1, CD_zero/1
  Sum/1 -> C_D/1
  CD_beta/1 -> Sum/3
  beta/1 -> CD_beta/1
  elevator_norm/1 -> Gain2/1
  posicao_do_flap/1 -> Gain3/1
  CD_zero/1 -> Scope2/1, Product1/2
  Product1/1 -> Gain4/1, Sum/1
  Gain1/1 -> Product2/2
  Product2/1 -> Sum/2, Gain6/1
  Ground-effect/1 -> Product4/1, Scope/1, Scope4/1, Product1/1, Product3/1, Product2/1
  Gain3/1 -> Product3/2
  Vel_mach/1 -> CD_mach/1
  CD_mach/1 -> Product4/2
  Product4/1 -> Sum/6
  Gain2/1 -> Sum/5
  Product3/1 -> Sum/4
  From Workspace9/1 -> Scope1/2
  Product5/1 -> Scope1/1
  Gain4/1 -> Product5/2
  Gain5/1 -> Ground-effect/1
  h/1 -> Gain5/1
  Gain6/1 -> Product6/2
  From Workspace2/1 -> Scope5/2
  Product6/1 -> Scope5/1
  qbar/1 -> Product6/1, Scope6/1, Product5/1
  From Workspace3/1 -> Gain7/1
  Gain7/1 -> Scope6/2

== system trim_cessna_t37/Aerodinamica/Forcas Aerodinamicas/Coef. Forca Lateral ==
  beta : Inport
  p : Inport  Port=2
  VT : Inport  Port=3
  r : Inport  Port=4
  rudder : Inport  Port=5
  Constant2 : Constant  Value=bw
  Gain : Gain  Gain=CY_rudder  SaturateOnIntegerOverflow=on  OutDataTypeStr=Inherit: Same as input  ParamDataTypeStr=Inherit: Same as input
  Gain1 : Gain  Gain=2  SaturateOnIntegerOverflow=on  OutDataTypeStr=Inherit: Same as input  ParamDataTypeStr=Inherit: Same as input
  Gain2 : Gain  Gain=CY_beta  SaturateOnIntegerOverflow=on  OutDataTypeStr=Inherit: Same as input  ParamDataTypeStr=Inherit: Same as input
  Gain3 : Gain  Gain=CY_p  SaturateOnIntegerOverflow=on  OutDataTypeStr=Inherit: Same as input  ParamDataTypeStr=Inherit: Same as input
  Gain4 : Gain  Gain=CY_r  SaturateOnIntegerOverflow=on  OutDataTypeStr=Inherit: Same as input  ParamDataTypeStr=Inherit: Same as input
  Product1 : Product  SaturateOnIntegerOverflow=on  OutDataTypeStr=Inherit: Same as first input
  Product2 : Product  SaturateOnIntegerOverflow=on  OutDataTypeStr=Inherit: Same as first input
  Product3 : Product  Inputs=*/  SaturateOnIntegerOverflow=on  OutDataTypeStr=Inherit: Same as first input
  Sum : Sum  Inputs=++++  SaturateOnIntegerOverflow=on
  C_Y : Outport
  wires:
  beta/1 -> Gain2/1
  Sum/1 -> C_Y/1
  Gain2/1 -> Sum/1
  Product1/1 -> Sum/2
  Gain3/1 -> Product1/1
  VT/1 -> Gain1/1
  Gain1/1 -> Product3/2
  Constant2/1 -> Product3/1
  Product3/1 -> Product1/2, Product2/1
  Product2/1 -> Sum/3
  r/1 -> Gain4/1
  Gain/1 -> Sum/4
  rudder/1 -> Gain/1
  Gain4/1 -> Product2/2
  p/1 -> Gain3/1

== system trim_cessna_t37/Aerodinamica/Forcas Aerodinamicas/Coef. sustentacao ==
  alpha : Inport
  alpha_dot : Inport  Port=2
  h : Inport  Port=3
  elevator : Inport  Port=4
  VT : Inport  Port=5
  q : Inport  Port=6
  "posicao_do_flap " : Inport  Port=7
  CL_alpha : Lookup  InputValues=CL_alpha(:,1);  Table=CL_alpha(:,2);  LookUpMeth=Interpolation-Use End Values  SaturateOnIntegerOverflow=on
  Constant2 : Constant  Value=cw
  Gain : Gain  Gain=1/bw  SaturateOnIntegerOverflow=on  OutDataTypeStr=Inherit: Same as input  ParamDataTypeStr=Inherit: Same as input
  Gain1 : Gain  Gain=2  SaturateOnIntegerOverflow=on  OutDataTypeStr=Inherit: Same as input  ParamDataTypeStr=Inherit: Same as input
  Gain2 : Gain  Gain=CL_q  SaturateOnIntegerOverflow=on  OutDataTypeStr=Inherit: Same as input  ParamDataTypeStr=Inherit: Same as input
  Gain3 : Gain  Gain=CL_elev  SaturateOnIntegerOverflow=on  OutDataTypeStr=Inherit: Same as input  ParamDataTypeStr=Inherit: Same as input
  Gain4 : Gain  Gain=CL_alpha_dot  SaturateOnIntegerOverflow=on  OutDataTypeStr=Inherit: Same as input  ParamDataTypeStr=Inherit: Same as input
  Gain5 : Gain  Gain=CL_flap  SaturateOnIntegerOverflow=on  OutDataTypeStr=Inherit: Same as input  ParamDataTypeStr=Inherit: Same as input
  Ground-effect : Lookup  InputValues=CL_ground_effect(:,1);  Table=CL_ground_effect(:,2);  LookUpMeth=Interpolation-Use End Values  SaturateOnIntegerOverflow=on
  Product{2,4..6} (4 alike) : Product  SaturateOnIntegerOverflow=on  OutDataTypeStr=Inherit: Same as first input
  Product3 : Product  Inputs=*/  SaturateOnIntegerOverflow=on  OutDataTypeStr=Inherit: Same as first input
  Sum1 : Sum  Inputs=+++++  SaturateOnIntegerOverflow=on
  C_L : Outport
  wires:
  alpha/1 -> CL_alpha/1
  Gain/1 -> Ground-effect/1
  h/1 -> Gain/1
  Sum1/1 -> C_L/1
  Gain4/1 -> Product2/1
  VT/1 -> Gain1/1
  Gain1/1 -> Product3/2
  Constant2/1 -> Product3/1
  Product2/1 -> Sum1/2
  Product3/1 -> Product2/2, Product4/2
  Gain2/1 -> Product4/1
  Product4/1 -> Sum1/3
  q/1 -> Gain2/1
  elevator/1 -> Gain3/1
  Gain3/1 -> Sum1/4
  alpha_dot/1 -> Gain4/1
  CL_alpha/1 -> Product5/1
  Ground-effect/1 -> Product5/2, Product6/2
  "posicao_do_flap "/1 -> Gain5/1
  Gain5/1 -> Product6/1
  Product5/1 -> Sum1/1
  Product6/1 -> Sum1/5

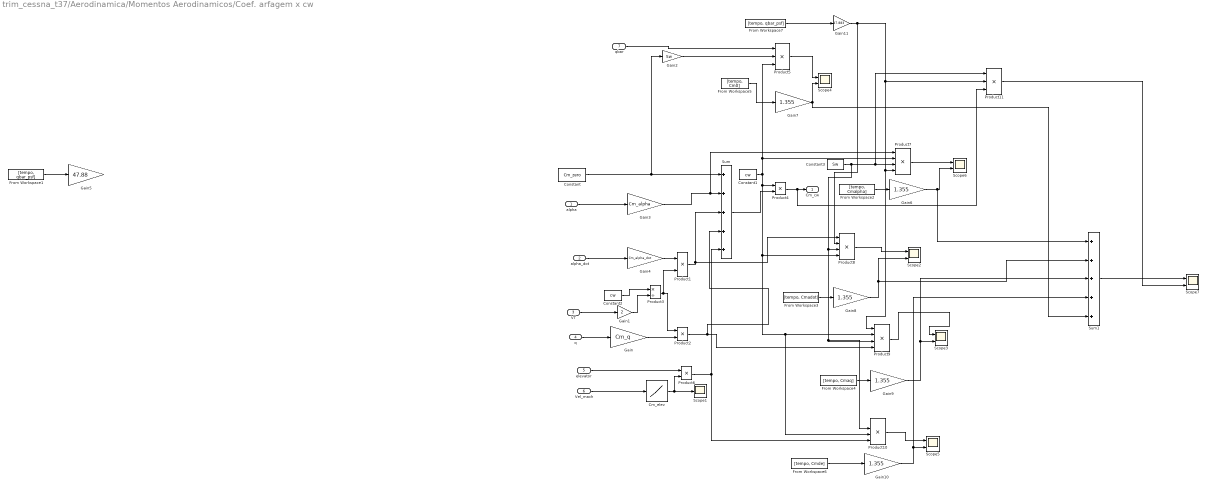
== system trim_cessna_t37/Aerodinamica/Momentos Aerodinamicos/Coef. arfagem x cw ==
  alpha : Inport
  alpha_dot : Inport  Port=2
  VT : Inport  Port=3
  q : Inport  Port=4
  elevator : Inport  Port=5
  Vel_mach : Inport  Port=6
  qbar : Inport  Port=7
  Cm_elev : Lookup  InputValues=Cm_elev(:,1);  Table=Cm_elev(:,2);  SaturateOnIntegerOverflow=on
  Constant : Constant  Value=Cm_zero
  Constant1 : Constant  Value=cw
  Constant2 : Constant  Value=cw
  Constant3 : Constant  Value=Sw
  From Workspace1 : FromWorkspace  VariableName=[tempo, qbar_psf]  SampleTime=0
  From Workspace2 : FromWorkspace  VariableName=[tempo, Cmalpha]  SampleTime=0
  From Workspace3 : FromWorkspace  VariableName=[tempo, Cmadot]  SampleTime=0
  From Workspace4 : FromWorkspace  VariableName=[tempo, Cmaq]  SampleTime=0
  From Workspace5 : FromWorkspace  VariableName=[tempo, Cm0]  SampleTime=0
  From Workspace6 : FromWorkspace  VariableName=[tempo, Cmde]  SampleTime=0
  From Workspace7 : FromWorkspace  VariableName=[tempo, qbar_psf]  SampleTime=0
  Gain : Gain  Gain=Cm_q  SaturateOnIntegerOverflow=on  OutDataTypeStr=Inherit: Same as input  ParamDataTypeStr=Inherit: Same as input
  Gain1 : Gain  Gain=2  SaturateOnIntegerOverflow=on  OutDataTypeStr=Inherit: Same as input  ParamDataTypeStr=Inherit: Same as input
  Gain{6..10} (5 alike) : Gain  Gain=1.355  SaturateOnIntegerOverflow=on  OutDataTypeStr=Inherit: Same as input  ParamDataTypeStr=Inherit: Same as input
  Gain11 : Gain  Gain=47.883  SaturateOnIntegerOverflow=on  OutDataTypeStr=Inherit: Same as input  ParamDataTypeStr=Inherit: Same as input
  Gain2 : Gain  Gain=Sw  SaturateOnIntegerOverflow=on  OutDataTypeStr=Inherit: Same as input  ParamDataTypeStr=Inherit: Same as input
  Gain3 : Gain  Gain=Cm_alpha  SaturateOnIntegerOverflow=on  OutDataTypeStr=Inherit: Same as input  ParamDataTypeStr=Inherit: Same as input
  Gain4 : Gain  Gain=Cm_alpha_dot  SaturateOnIntegerOverflow=on  OutDataTypeStr=Inherit: Same as input  ParamDataTypeStr=Inherit: Same as input
  Gain5 : Gain  Gain=47.88  SaturateOnIntegerOverflow=on  OutDataTypeStr=Inherit: Same as input  ParamDataTypeStr=Inherit: Same as input
  Product{1..2,4,6} (4 alike) : Product  Inputs=**  SaturateOnIntegerOverflow=on  OutDataTypeStr=Inherit: Same as first input
  Product{7..10} (4 alike) : Product  Inputs=****  SaturateOnIntegerOverflow=on  OutDataTypeStr=Inherit: Same as first input
  Product11 : Product  Inputs=***  SaturateOnIntegerOverflow=on  OutDataTypeStr=Inherit: Same as first input
  Product3 : Product  Inputs=*/  SaturateOnIntegerOverflow=on  OutDataTypeStr=Inherit: Same as first input
  Product5 : Product  Inputs=***  SaturateOnIntegerOverflow=on  OutDataTypeStr=Inherit: Same as first input
  Scope1 : Scope
  Scope{2..7} (6 alike) : Scope  NumInputPorts=2
  Sum : Sum  Inputs=+++++  SaturateOnIntegerOverflow=on
  Sum1 : Sum  Inputs=+++++  SaturateOnIntegerOverflow=on
  Cm_cw : Outport
  wires:
  alpha/1 -> Gain3/1
  Constant1/1 -> Product5/3, Product7/2, Product10/3, Product9/2, Product8/4, Product4/1
  Sum/1 -> Product4/2
  VT/1 -> Gain1/1
  Gain1/1 -> Product3/2
  Constant2/1 -> Product3/1
  q/1 -> Gain/1
  Gain/1 -> Product2/2
  Gain3/1 -> Product7/1, Sum/2
  Gain4/1 -> Product1/1
  alpha_dot/1 -> Gain4/1
  Product3/1 -> Product2/1, Product1/2
  elevator/1 -> Product6/1
  Cm_elev/1 -> Scope1/1, Product6/2
  Product6/1 -> Sum/5, Product10/4
  Vel_mach/1 -> Cm_elev/1
  Gain2/1 -> Product5/2
  Product5/1 -> Scope4/1
  Constant3/1 -> Product10/2, Product9/3, Product8/3, Product11/1, Product7/3
  Product7/1 -> Scope6/1
  From Workspace1/1 -> Gain5/1
  qbar/1 -> Product5/1
  Constant/1 -> Gain2/1, Sum/1
  From Workspace2/1 -> Gain6/1
  Gain6/1 -> Sum1/1, Scope6/2
  From Workspace5/1 -> Gain7/1
  Gain7/1 -> Scope4/2, Sum1/5
  From Workspace3/1 -> Gain8/1
  Product1/1 -> Product8/1, Sum/3
  Gain8/1 -> Sum1/2, Scope2/2
  Product8/1 -> Scope2/1
  From Workspace4/1 -> Gain9/1
  Gain9/1 -> Sum1/3, Scope3/2
  Product9/1 -> Scope3/1
  Product2/1 -> Sum/4, Product9/4
  Product10/1 -> Scope5/1
  From Workspace6/1 -> Gain10/1
  Gain10/1 -> Sum1/4, Scope5/2
  Sum1/1 -> Scope7/1
  Product4/1 -> Product11/3, Cm_cw/1
  Product11/1 -> Scope7/2
  From Workspace7/1 -> Gain11/1
  Gain11/1 -> Product8/2, Product11/2, Product9/1, Product7/4

== system trim_cessna_t37/Aerodinamica/Momentos Aerodinamicos/Coef. guinada x bw ==
  beta : Inport
  p : Inport  Port=2
  VT : Inport  Port=3
  r : Inport  Port=4
  rudder : Inport  Port=5
  "aileron " : Inport  Port=6
  Constant1 : Constant  Value=bw
  Constant2 : Constant  Value=bw
  Gain1 : Gain  Gain=2  SaturateOnIntegerOverflow=on  OutDataTypeStr=Inherit: Same as input  ParamDataTypeStr=Inherit: Same as input
  Gain2 : Gain  Gain=Cn_p  SaturateOnIntegerOverflow=on  OutDataTypeStr=Inherit: Same as input  ParamDataTypeStr=Inherit: Same as input
  Gain3 : Gain  Gain=Cn_beta  SaturateOnIntegerOverflow=on  OutDataTypeStr=Inherit: Same as input  ParamDataTypeStr=Inherit: Same as input
  Gain4 : Gain  Gain=Cn_r  SaturateOnIntegerOverflow=on  OutDataTypeStr=Inherit: Same as input  ParamDataTypeStr=Inherit: Same as input
  Gain5 : Gain  Gain=Cn_rudder  SaturateOnIntegerOverflow=on  OutDataTypeStr=Inherit: Same as input  ParamDataTypeStr=Inherit: Same as input
  Gain6 : Gain  Gain=Cnda  SaturateOnIntegerOverflow=on  OutDataTypeStr=Inherit: Same as input  ParamDataTypeStr=Inherit: Same as input
  Gain7 : Gain  Gain=DCnpDf  SaturateOnIntegerOverflow=on  OutDataTypeStr=Inherit: Same as input  ParamDataTypeStr=Inherit: Same as input
  Product{1..2,4,6} (4 alike) : Product  Inputs=**  SaturateOnIntegerOverflow=on  OutDataTypeStr=Inherit: Same as first input
  Product3 : Product  Inputs=*/  SaturateOnIntegerOverflow=on  OutDataTypeStr=Inherit: Same as first input
  Sum : Sum  Inputs=++++++  SaturateOnIntegerOverflow=on
  Cn_bw : Outport
  wires:
  Constant1/1 -> Product4/1
  Sum/1 -> Product4/2
  Product4/1 -> Cn_bw/1
  VT/1 -> Gain1/1
  Gain1/1 -> Product3/2
  Constant2/1 -> Product3/1
  beta/1 -> Gain3/1
  Gain3/1 -> Sum/1
  Product3/1 -> Product2/2, Product1/2, Product6/1
  Product1/1 -> Sum/2
  r/1 -> Gain4/1
  Product6/1 -> Sum/3
  rudder/1 -> Gain5/1
  Gain2/1 -> Product1/1
  Gain4/1 -> Product6/2
  Gain5/1 -> Sum/4
  p/1 -> Gain7/1, Gain2/1
  "aileron "/1 -> Gain6/1
  Gain6/1 -> Sum/5
  Gain7/1 -> Product2/1
  Product2/1 -> Sum/6

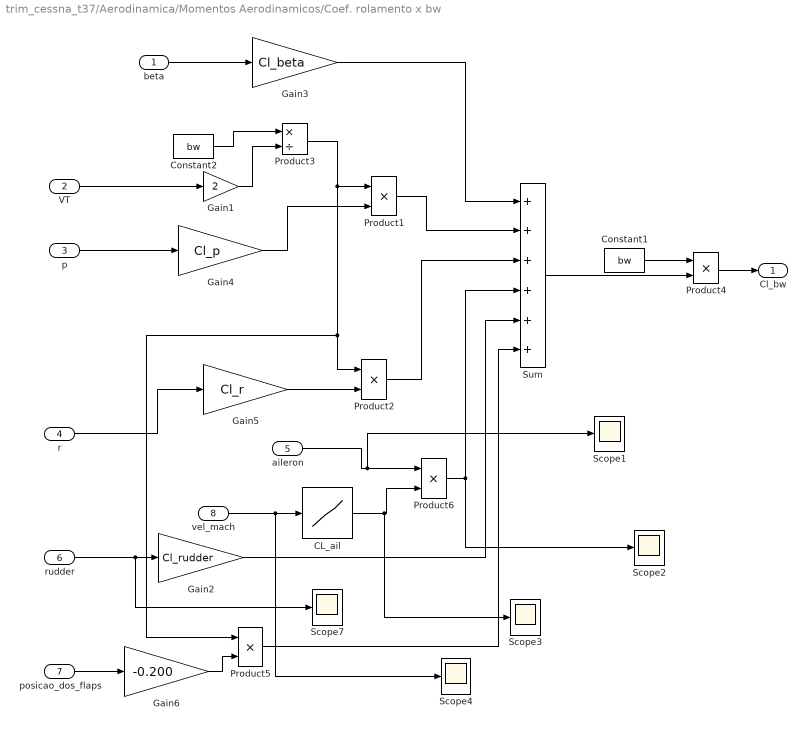
== system trim_cessna_t37/Aerodinamica/Momentos Aerodinamicos/Coef. rolamento x bw ==
  beta : Inport
  VT : Inport  Port=2
  p : Inport  Port=3
  r : Inport  Port=4
  aileron : Inport  Port=5
  rudder : Inport  Port=6
  posicao_dos_flaps : Inport  Port=7
  vel_mach : Inport  Port=8
  CL_ail : Lookup  InputValues=Cl_ail(:,1);  Table=Cl_ail(:,2);  SaturateOnIntegerOverflow=on
  Constant1 : Constant  Value=bw
  Constant2 : Constant  Value=bw
  Gain1 : Gain  Gain=2  SaturateOnIntegerOverflow=on  OutDataTypeStr=Inherit: Same as input  ParamDataTypeStr=Inherit: Same as input
  Gain2 : Gain  Gain=Cl_rudder  SaturateOnIntegerOverflow=on  OutDataTypeStr=Inherit: Same as input  ParamDataTypeStr=Inherit: Same as input
  Gain3 : Gain  Gain=Cl_beta  SaturateOnIntegerOverflow=on  OutDataTypeStr=Inherit: Same as input  ParamDataTypeStr=Inherit: Same as input
  Gain4 : Gain  Gain=Cl_p  SaturateOnIntegerOverflow=on  OutDataTypeStr=Inherit: Same as input  ParamDataTypeStr=Inherit: Same as input
  Gain5 : Gain  Gain=Cl_r  SaturateOnIntegerOverflow=on  OutDataTypeStr=Inherit: Same as input  ParamDataTypeStr=Inherit: Same as input
  Gain6 : Gain  Gain=-0.200  SaturateOnIntegerOverflow=on  OutDataTypeStr=Inherit: Same as input  ParamDataTypeStr=Inherit: Same as input
  Product{1..2,5..6} (4 alike) : Product  SaturateOnIntegerOverflow=on  OutDataTypeStr=Inherit: Same as first input
  Product3 : Product  Inputs=*/  SaturateOnIntegerOverflow=on  OutDataTypeStr=Inherit: Same as first input
  Product4 : Product  Inputs=**  SaturateOnIntegerOverflow=on  OutDataTypeStr=Inherit: Same as first input
  Scope{1..4,7} (5 alike) : Scope
  Sum : Sum  Inputs=++++++  SaturateOnIntegerOverflow=on
  Cl_bw : Outport
  wires:
  VT/1 -> Gain1/1
  Gain1/1 -> Product3/2
  Constant2/1 -> Product3/1
  Product3/1 -> Product1/1, Product5/1, Product2/1
  Gain4/1 -> Product1/2
  r/1 -> Gain5/1
  rudder/1 -> Scope7/1, Gain2/1
  Product1/1 -> Sum/2
  Product2/1 -> Sum/3
  Gain2/1 -> Sum/5
  Constant1/1 -> Product4/1
  Sum/1 -> Product4/2
  Product4/1 -> Cl_bw/1
  Gain5/1 -> Product2/2
  Gain3/1 -> Sum/1
  p/1 -> Gain4/1
  Gain6/1 -> Product5/2
  posicao_dos_flaps/1 -> Gain6/1
  beta/1 -> Gain3/1
  vel_mach/1 -> Scope4/1, CL_ail/1
  aileron/1 -> Scope1/1, Product6/1
  CL_ail/1 -> Scope3/1, Product6/2
  Product6/1 -> Sum/4, Scope2/1
  Product5/1 -> Sum/6
